simulink model "visualise"  (R2020a)
settings: Solver=FixedStepAuto  StartTime=0.0  StopTime=inf  FixedStep=1/simVars.visFreq  RelTol=1e-3
InitFcn:
  | vis_init
undefined symbols (not defined in the file): simVars
settings Model: Creator=Matthias  LastModifiedBy=sihao
settings DataIOCC: ReturnWorkspaceOutputs=off
settings DebuggingCC: ArithmeticOperatorsInVariantConditions=warning
settings SFSimCC: CustomCodeUndefinedFunction=UseInterfaceOnly

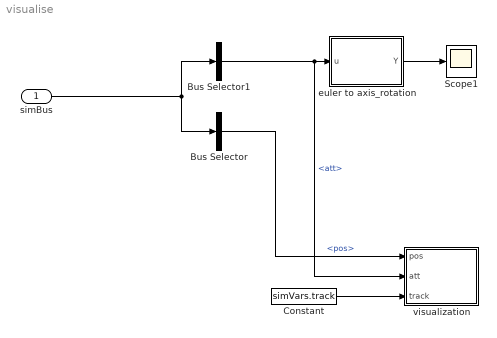
== system visualise ==
  simBus : Inport  OutDataTypeStr=Bus: simBus
  Bus Selector : BusSelector  OutputSignals=pos
  Bus Selector1 : BusSelector  OutputSignals=att
  Constant : Constant  Value=simVars.track
  Scope1 : Scope
  euler to axis_rotation : MATLAB Function  TreatAsAtomicUnit=on
  visualization : MATLAB Function  TreatAsAtomicUnit=on
  wires:
  Bus Selector1/1 -> visualization/2(att), euler to axis_rotation/1(u)  "<att>"
  euler to axis_rotation/1(Y) -> Scope1/1
  Bus Selector/1 -> visualization/1(pos)  "<pos>"
  simBus/1 -> Bus Selector/1, Bus Selector1/1
  Constant/1 -> visualization/3(track)

== matlab function visualise/visualization ==
  settings: updateMethod=DISCRETE  sampleTime=1/simVars.visFreq
  data: pos input; att input; track input
function fcn(pos,att,track)

persistent posTrack; if isempty(posTrack); posTrack = [pos(1),pos(2),pos(3)]; end

x = pos(1);
y = pos(2);
z = pos(3);

posTrack = [posTrack; [pos(1),pos(2),pos(3)]];

phi = att(1);
theta = att(2);
yaw = att(3);


% Drone
t = get(gca,'Children');
t = t(2);

S = makehgtform('translate',[x y z]);
Rz = makehgtform('zrotate',yaw);
Ry = makehgtform('yrotate',theta);
Rx = makehgtform('xrotate',phi);

set(t,'Matrix',S*Rz*Ry*Rx);
% set(t,'Matrix',S);

% trajectory
t = get(gca,'Children');
t = t(1);
set(t, 'XData', posTrack(:,1));
set(t, 'YData', posTrack(:,2));
set(t, 'ZData', posTrack(:,3));

drawnow

if track
   xlim([x-2.5,x+1.5]); ylim([y-2,y+2]); zlim([z-2,z+2]);
else
   xlim([-2.5,1.5]); ylim([-2,2]); zlim([-2,2])
end

end

== matlab function visualise/euler to axis_rotation ==
  data: u input; Y output
function Y = euler_axisrotation(u)
%#codegen
% 
phi = u(1);
theta = u(2);
psi = u(3);
% 
% c1 = cos(psi/2);
% c2 = cos(theta/2);
% c3 = cos(phi/2);
% 
% s1 = sin(psi/2);
% s2 = sin(theta/2);
% s3 = sin(phi/2);
% 
% angle = 2*acos(c1*c2*c3-s1*s2*s3);
% x = s1*s2*c3+c1*c2*s3;
% y = s1*c2*c3+c1*s2*s3;
% z = c1*s2*c3-s1*c2*s3;
% x = x/norm([x y z]);
% y = y/norm([x y z]);
% z = z/norm([x y z]);
% 
% eul = [psi theta phi];
q = angle2quat_diy(psi,theta,phi);
qw = q(1); qx = q(2); qy = q(3); qz = q(4);
angle = 2*acos(qw);
x = qx/sqrt(1-qw^2);
y = qy/sqrt(1-qw^2);
z = qz/sqrt(1-qw^2);

Y = [x y z angle];
end


function q = angle2quat_diy( r1, r2, r3 )

angles = [r1(:) r2(:) r3(:)];

cang = cos( angles/2 );
sang = sin( angles/2 );

q = [ cang(:,1).*cang(:,2).*cang(:,3) + sang(:,1).*sang(:,2).*sang(:,3), ...
    cang(:,1).*cang(:,2).*sang(:,3) - sang(:,1).*sang(:,2).*cang(:,3), ...
    cang(:,1).*sang(:,2).*cang(:,3) + sang(:,1).*cang(:,2).*sang(:,3), ...
    sang(:,1).*cang(:,2).*cang(:,3) - cang(:,1).*sang(:,2).*sang(:,3)];

end
